simulink model "ctrl_student_HIL103007042017"  (R2015a)
settings: Solver=ode3  StartTime=0.0  StopTime=inf  FixedStep=0.01  RelTol=1e-3
values from neighbouring files (symbols this model uses):
  DesiredPath = 0    [Innput.m]    (also in Input_v3.m = 1)
  Elipscenter_radi = [6 5;0 3 ]    [Innput.m]    (also in Input_v3.m = [3 2;0 1 ])
  eta_dot_ini = [7;0;0]    [Innput.m]    (also in Input_v3.m)
  K = [2;10]    [Input_v3.m]
  K1 = diag([1,1,4])    [Input_v3.m]
  K2 = diag([200,50,3])    [Input_v3.m]    (also in inputDPgains.m = [1 0 0; 0 1 0; 0 0 1])
  l1 = [1 0 0;0 1 0;0 0 0.05]    [Input_v3.m]    (also in inputDPgains.m = [1 0 0; 0 1 0; 0 0 1])
  l2 = [1 0 0;0 1 0;0 0 0.05]    [Input_v3.m]    (also in inputDPgains.m = [1 0 0; 0 1 0; 0 0 1])
  l3 = [1 0 0;0 1 0;0 0 0.05]    [Input_v3.m]    (also in inputDPgains.m = [1 0 0; 0 1 0; 0 0 1])
  LAW = 1    [Innput.m]    (also in Input_v3.m = 0)
  lim = [1.00;-20;6.45/2;-6.45/2]    [Innput.m]    (also in Input_v3.m = [20;-20;9;-9])
  lim_2 = [1.5;-22;7;-7]    [Innput.m]    (also in Input_v3.m = [25;-25;10;-10])
  m = 14.79    [Input_v3.m]    (also in ctrl_student_init.m)
  mu = mu(1)    [Innput.m]    (also in Input_v3.m = 0.001)
  pd = [2 10;0 4]    [Input_v3.m]
  T_initialDP = T_initialDP*100    (= 6000)    [Input_v3.m]
  U_ref = 0.1    [Innput.m]    (also in Input_v3.m)
libraries: simulink x2
(part 3 of 5)

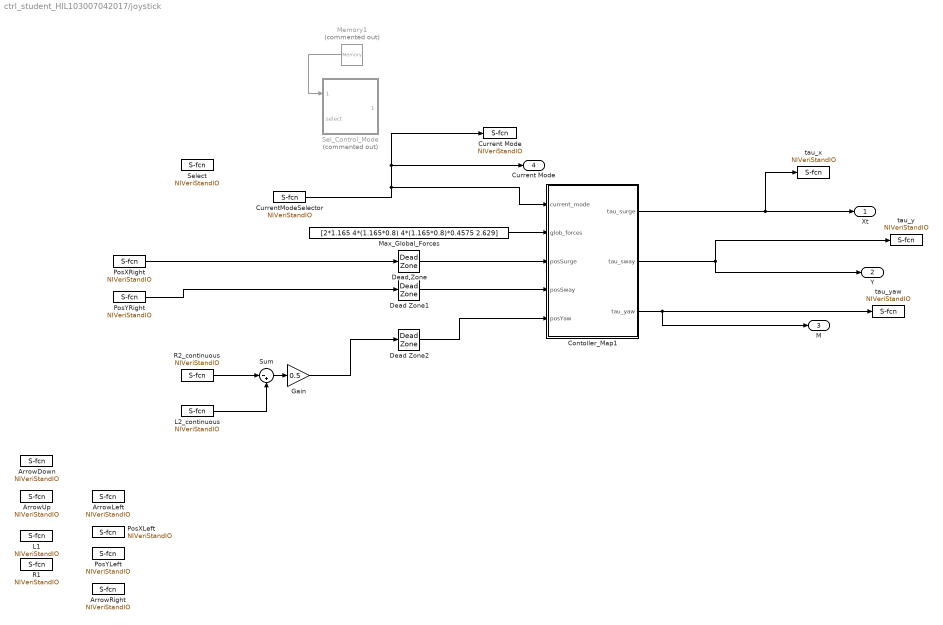
== system ctrl_student_HIL103007042017/joystick ==
  ArrowDown : S-Function  Priority=9  FunctionName=NIVeriStandIO  Parameters=width dtype portnum stime stype btype  mask(NI VeriStand Inport){portnum=9, width=-1, stime=-1, dtype=auto, stype=auto, btype=1}
      mask prompts: portnum "Port number:"; width "Port dimensions (-1 for dynamically sized):"; stime "Sample time (-1 for inherited):"; dtype "Data type:"; stype "Signal type:"; btype "Block type:"
      mask help: Use this inport on any level of nested subsystems to allow NI VeriStand software to map signals to it.
      mask init:
      | NIVeriStandIO_init;
      settings: CopyFcn=NIVeriStand_MDL_functions('', 'IO_copy');  DeleteFcn=NIVeriStand_MDL_functions('', 'IO_delete');  MoveFcn=set_param(gcb, 'Mask', 'on');
      mask Callback portnum: NIVeriStand_MDL_functions('', 'IO_setportnum');
      mask TypeOptions dtype: auto | double | single | int8 | uint8 | int16 | uint16 | int32 | uint32 | boolean
      mask Callback dtype: NIVeriStand_MDL_functions('', 'IO_booleansignal');
      mask TypeOptions stype: auto | real | complex
      mask Display:
      | patch([-x x], [-y y], [.90980 .81960 .32156]);
      | plot([xrad -x x xrad], [yrad -y y yrad]);
      | fprintf('NI In%d', portnum);
  ArrowLeft : S-Function  Priority=11  FunctionName=NIVeriStandIO  Parameters=width dtype portnum stime stype btype  mask(NI VeriStand Inport){portnum=11, width=-1, stime=-1, dtype=auto, stype=auto, btype=1}
      mask prompts: portnum "Port number:"; width "Port dimensions (-1 for dynamically sized):"; stime "Sample time (-1 for inherited):"; dtype "Data type:"; stype "Signal type:"; btype "Block type:"
      mask help: Use this inport on any level of nested subsystems to allow NI VeriStand software to map signals to it.
      mask init:
      | NIVeriStandIO_init;
      settings: CopyFcn=NIVeriStand_MDL_functions('', 'IO_copy');  DeleteFcn=NIVeriStand_MDL_functions('', 'IO_delete');  MoveFcn=set_param(gcb, 'Mask', 'on');
      mask Callback portnum: NIVeriStand_MDL_functions('', 'IO_setportnum');
      mask TypeOptions dtype: auto | double | single | int8 | uint8 | int16 | uint16 | int32 | uint32 | boolean
      mask Callback dtype: NIVeriStand_MDL_functions('', 'IO_booleansignal');
      mask TypeOptions stype: auto | real | complex
      mask Display:
      | patch([-x x], [-y y], [.90980 .81960 .32156]);
      | plot([xrad -x x xrad], [yrad -y y yrad]);
      | fprintf('NI In%d', portnum);
  ArrowRight : S-Function  Priority=12  FunctionName=NIVeriStandIO  Parameters=width dtype portnum stime stype btype  mask(NI VeriStand Inport){portnum=12, width=-1, stime=-1, dtype=auto, stype=auto, btype=1}
      mask prompts: portnum "Port number:"; width "Port dimensions (-1 for dynamically sized):"; stime "Sample time (-1 for inherited):"; dtype "Data type:"; stype "Signal type:"; btype "Block type:"
      mask help: Use this inport on any level of nested subsystems to allow NI VeriStand software to map signals to it.
      mask init:
      | NIVeriStandIO_init;
      settings: CopyFcn=NIVeriStand_MDL_functions('', 'IO_copy');  DeleteFcn=NIVeriStand_MDL_functions('', 'IO_delete');  MoveFcn=set_param(gcb, 'Mask', 'on');
      mask Callback portnum: NIVeriStand_MDL_functions('', 'IO_setportnum');
      mask TypeOptions dtype: auto | double | single | int8 | uint8 | int16 | uint16 | int32 | uint32 | boolean
      mask Callback dtype: NIVeriStand_MDL_functions('', 'IO_booleansignal');
      mask TypeOptions stype: auto | real | complex
      mask Display:
      | patch([-x x], [-y y], [.90980 .81960 .32156]);
      | plot([xrad -x x xrad], [yrad -y y yrad]);
      | fprintf('NI In%d', portnum);
  ArrowUp : S-Function  Priority=10  FunctionName=NIVeriStandIO  Parameters=width dtype portnum stime stype btype  mask(NI VeriStand Inport){portnum=10, width=-1, stime=-1, dtype=auto, stype=auto, btype=1}
      mask prompts: portnum "Port number:"; width "Port dimensions (-1 for dynamically sized):"; stime "Sample time (-1 for inherited):"; dtype "Data type:"; stype "Signal type:"; btype "Block type:"
      mask help: Use this inport on any level of nested subsystems to allow NI VeriStand software to map signals to it.
      mask init:
      | NIVeriStandIO_init;
      settings: CopyFcn=NIVeriStand_MDL_functions('', 'IO_copy');  DeleteFcn=NIVeriStand_MDL_functions('', 'IO_delete');  MoveFcn=set_param(gcb, 'Mask', 'on');
      mask Callback portnum: NIVeriStand_MDL_functions('', 'IO_setportnum');
      mask TypeOptions dtype: auto | double | single | int8 | uint8 | int16 | uint16 | int32 | uint32 | boolean
      mask Callback dtype: NIVeriStand_MDL_functions('', 'IO_booleansignal');
      mask TypeOptions stype: auto | real | complex
      mask Display:
      | patch([-x x], [-y y], [.90980 .81960 .32156]);
      | plot([xrad -x x xrad], [yrad -y y yrad]);
      | fprintf('NI In%d', portnum);
  Contoller_Map1 : MATLAB Function  TreatAsAtomicUnit=on
  "Current Mode " : S-Function  Priority=1  FunctionName=NIVeriStandIO  Parameters=width dtype portnum stime stype btype  mask(NI VeriStand Outport){portnum=1, width=-1, stime=-1, dtype=auto, stype=auto, btype=0}
      mask prompts: portnum "Port number:"; width "Port dimensions (-1 for dynamically sized):"; stime "Sample time (-1 for inherited):"; dtype "Data type:"; stype "Signal type:"; btype "Block type:"
      mask help: Use this outport on any level of nested subsystems to allow NI VeriStand software to map signals to it.
      mask init:
      | NIVeriStandIO_init;
      settings: CopyFcn=NIVeriStand_MDL_functions('', 'IO_copy');  DeleteFcn=NIVeriStand_MDL_functions('', 'IO_delete');  MoveFcn=set_param(gcb, 'Mask', 'on');
      mask Callback portnum: NIVeriStand_MDL_functions('', 'IO_setportnum');
      mask TypeOptions dtype: auto | double | single | int8 | uint8 | int16 | uint16 | int32 | uint32 | boolean
      mask Callback dtype: NIVeriStand_MDL_functions('', 'IO_booleansignal');
      mask TypeOptions stype: auto | real | complex
      mask Display:
      | patch([-x x], [-y y], [.90980 .81960 .32156]);
      | plot([xrad -x x xrad], [yrad -y y yrad]);
      | fprintf('NI Out%d', portnum);
  CurrentModeSelector : S-Function  Priority=14  FunctionName=NIVeriStandIO  Parameters=width dtype portnum stime stype btype  mask(NI VeriStand Inport){portnum=14, width=-1, stime=-1, dtype=auto, stype=auto, btype=1}
      mask prompts: portnum "Port number:"; width "Port dimensions (-1 for dynamically sized):"; stime "Sample time (-1 for inherited):"; dtype "Data type:"; stype "Signal type:"; btype "Block type:"
      mask help: Use this inport on any level of nested subsystems to allow NI VeriStand software to map signals to it.
      mask init:
      | NIVeriStandIO_init;
      settings: CopyFcn=NIVeriStand_MDL_functions('', 'IO_copy');  DeleteFcn=NIVeriStand_MDL_functions('', 'IO_delete');  MoveFcn=set_param(gcb, 'Mask', 'on');
      mask Callback portnum: NIVeriStand_MDL_functions('', 'IO_setportnum');
      mask TypeOptions dtype: auto | double | single | int8 | uint8 | int16 | uint16 | int32 | uint32 | boolean
      mask Callback dtype: NIVeriStand_MDL_functions('', 'IO_booleansignal');
      mask TypeOptions stype: auto | real | complex
      mask Display:
      | patch([-x x], [-y y], [.90980 .81960 .32156]);
      | plot([xrad -x x xrad], [yrad -y y yrad]);
      | fprintf('NI In%d', portnum);
  Dead Zone : DeadZone  LowerValue=-0.05  UpperValue=0.05  SaturateOnIntegerOverflow=on
  Dead Zone1 : DeadZone  LowerValue=-0.05  UpperValue=0.05  SaturateOnIntegerOverflow=on
  Dead Zone2 : DeadZone  LowerValue=-0.05  UpperValue=0.05  SaturateOnIntegerOverflow=on
  Gain : Gain  Gain=0.5
  L1 : S-Function  Priority=7  FunctionName=NIVeriStandIO  Parameters=width dtype portnum stime stype btype  mask(NI VeriStand Inport){portnum=7, width=-1, stime=-1, dtype=auto, stype=auto, btype=1}
      mask prompts: portnum "Port number:"; width "Port dimensions (-1 for dynamically sized):"; stime "Sample time (-1 for inherited):"; dtype "Data type:"; stype "Signal type:"; btype "Block type:"
      mask help: Use this inport on any level of nested subsystems to allow NI VeriStand software to map signals to it.
      mask init:
      | NIVeriStandIO_init;
      settings: CopyFcn=NIVeriStand_MDL_functions('', 'IO_copy');  DeleteFcn=NIVeriStand_MDL_functions('', 'IO_delete');  MoveFcn=set_param(gcb, 'Mask', 'on');
      mask Callback portnum: NIVeriStand_MDL_functions('', 'IO_setportnum');
      mask TypeOptions dtype: auto | double | single | int8 | uint8 | int16 | uint16 | int32 | uint32 | boolean
      mask Callback dtype: NIVeriStand_MDL_functions('', 'IO_booleansignal');
      mask TypeOptions stype: auto | real | complex
      mask Display:
      | patch([-x x], [-y y], [.90980 .81960 .32156]);
      | plot([xrad -x x xrad], [yrad -y y yrad]);
      | fprintf('NI In%d', portnum);
  L2_continuous : S-Function  Priority=1  FunctionName=NIVeriStandIO  Parameters=width dtype portnum stime stype btype  mask(NI VeriStand Inport){portnum=1, width=-1, stime=-1, dtype=auto, stype=auto, btype=1}
      mask prompts: portnum "Port number:"; width "Port dimensions (-1 for dynamically sized):"; stime "Sample time (-1 for inherited):"; dtype "Data type:"; stype "Signal type:"; btype "Block type:"
      mask help: Use this inport on any level of nested subsystems to allow NI VeriStand software to map signals to it.
      mask init:
      | NIVeriStandIO_init;
      settings: CopyFcn=NIVeriStand_MDL_functions('', 'IO_copy');  DeleteFcn=NIVeriStand_MDL_functions('', 'IO_delete');  MoveFcn=set_param(gcb, 'Mask', 'on');
      mask Callback portnum: NIVeriStand_MDL_functions('', 'IO_setportnum');
      mask TypeOptions dtype: auto | double | single | int8 | uint8 | int16 | uint16 | int32 | uint32 | boolean
      mask Callback dtype: NIVeriStand_MDL_functions('', 'IO_booleansignal');
      mask TypeOptions stype: auto | real | complex
      mask Display:
      | patch([-x x], [-y y], [.90980 .81960 .32156]);
      | plot([xrad -x x xrad], [yrad -y y yrad]);
      | fprintf('NI In%d', portnum);
  Max_Global_Forces : Constant  Value=[2*1.165 4*(1.165*0.8) 4*(1.165*0.8)*0.4575 2.629]
  Memory1 : Memory  Commented=on  X0=2
  PosXLeft : S-Function  Priority=5  FunctionName=NIVeriStandIO  Parameters=width dtype portnum stime stype btype  mask(NI VeriStand Inport){portnum=5, width=-1, stime=-1, dtype=auto, stype=auto, btype=1}
      mask prompts: portnum "Port number:"; width "Port dimensions (-1 for dynamically sized):"; stime "Sample time (-1 for inherited):"; dtype "Data type:"; stype "Signal type:"; btype "Block type:"
      mask help: Use this inport on any level of nested subsystems to allow NI VeriStand software to map signals to it.
      mask init:
      | NIVeriStandIO_init;
      settings: CopyFcn=NIVeriStand_MDL_functions('', 'IO_copy');  DeleteFcn=NIVeriStand_MDL_functions('', 'IO_delete');  MoveFcn=set_param(gcb, 'Mask', 'on');
      mask Callback portnum: NIVeriStand_MDL_functions('', 'IO_setportnum');
      mask TypeOptions dtype: auto | double | single | int8 | uint8 | int16 | uint16 | int32 | uint32 | boolean
      mask Callback dtype: NIVeriStand_MDL_functions('', 'IO_booleansignal');
      mask TypeOptions stype: auto | real | complex
      mask Display:
      | patch([-x x], [-y y], [.90980 .81960 .32156]);
      | plot([xrad -x x xrad], [yrad -y y yrad]);
      | fprintf('NI In%d', portnum);
  PosXRight : S-Function  Priority=2  FunctionName=NIVeriStandIO  Parameters=width dtype portnum stime stype btype  mask(NI VeriStand Inport){portnum=2, width=-1, stime=-1, dtype=auto, stype=auto, btype=1}
      mask prompts: portnum "Port number:"; width "Port dimensions (-1 for dynamically sized):"; stime "Sample time (-1 for inherited):"; dtype "Data type:"; stype "Signal type:"; btype "Block type:"
      mask help: Use this inport on any level of nested subsystems to allow NI VeriStand software to map signals to it.
      mask init:
      | NIVeriStandIO_init;
      settings: CopyFcn=NIVeriStand_MDL_functions('', 'IO_copy');  DeleteFcn=NIVeriStand_MDL_functions('', 'IO_delete');  MoveFcn=set_param(gcb, 'Mask', 'on');
      mask Callback portnum: NIVeriStand_MDL_functions('', 'IO_setportnum');
      mask TypeOptions dtype: auto | double | single | int8 | uint8 | int16 | uint16 | int32 | uint32 | boolean
      mask Callback dtype: NIVeriStand_MDL_functions('', 'IO_booleansignal');
      mask TypeOptions stype: auto | real | complex
      mask Display:
      | patch([-x x], [-y y], [.90980 .81960 .32156]);
      | plot([xrad -x x xrad], [yrad -y y yrad]);
      | fprintf('NI In%d', portnum);
  PosYLeft : S-Function  Priority=6  FunctionName=NIVeriStandIO  Parameters=width dtype portnum stime stype btype  mask(NI VeriStand Inport){portnum=6, width=-1, stime=-1, dtype=auto, stype=auto, btype=1}
      mask prompts: portnum "Port number:"; width "Port dimensions (-1 for dynamically sized):"; stime "Sample time (-1 for inherited):"; dtype "Data type:"; stype "Signal type:"; btype "Block type:"
      mask help: Use this inport on any level of nested subsystems to allow NI VeriStand software to map signals to it.
      mask init:
      | NIVeriStandIO_init;
      settings: CopyFcn=NIVeriStand_MDL_functions('', 'IO_copy');  DeleteFcn=NIVeriStand_MDL_functions('', 'IO_delete');  MoveFcn=set_param(gcb, 'Mask', 'on');
      mask Callback portnum: NIVeriStand_MDL_functions('', 'IO_setportnum');
      mask TypeOptions dtype: auto | double | single | int8 | uint8 | int16 | uint16 | int32 | uint32 | boolean
      mask Callback dtype: NIVeriStand_MDL_functions('', 'IO_booleansignal');
      mask TypeOptions stype: auto | real | complex
      mask Display:
      | patch([-x x], [-y y], [.90980 .81960 .32156]);
      | plot([xrad -x x xrad], [yrad -y y yrad]);
      | fprintf('NI In%d', portnum);
  PosYRight : S-Function  Priority=3  FunctionName=NIVeriStandIO  Parameters=width dtype portnum stime stype btype  mask(NI VeriStand Inport){portnum=3, width=-1, stime=-1, dtype=auto, stype=auto, btype=1}
      mask prompts: portnum "Port number:"; width "Port dimensions (-1 for dynamically sized):"; stime "Sample time (-1 for inherited):"; dtype "Data type:"; stype "Signal type:"; btype "Block type:"
      mask help: Use this inport on any level of nested subsystems to allow NI VeriStand software to map signals to it.
      mask init:
      | NIVeriStandIO_init;
      settings: CopyFcn=NIVeriStand_MDL_functions('', 'IO_copy');  DeleteFcn=NIVeriStand_MDL_functions('', 'IO_delete');  MoveFcn=set_param(gcb, 'Mask', 'on');
      mask Callback portnum: NIVeriStand_MDL_functions('', 'IO_setportnum');
      mask TypeOptions dtype: auto | double | single | int8 | uint8 | int16 | uint16 | int32 | uint32 | boolean
      mask Callback dtype: NIVeriStand_MDL_functions('', 'IO_booleansignal');
      mask TypeOptions stype: auto | real | complex
      mask Display:
      | patch([-x x], [-y y], [.90980 .81960 .32156]);
      | plot([xrad -x x xrad], [yrad -y y yrad]);
      | fprintf('NI In%d', portnum);
  R1 : S-Function  Priority=8  FunctionName=NIVeriStandIO  Parameters=width dtype portnum stime stype btype  mask(NI VeriStand Inport){portnum=8, width=-1, stime=-1, dtype=auto, stype=auto, btype=1}
      mask prompts: portnum "Port number:"; width "Port dimensions (-1 for dynamically sized):"; stime "Sample time (-1 for inherited):"; dtype "Data type:"; stype "Signal type:"; btype "Block type:"
      mask help: Use this inport on any level of nested subsystems to allow NI VeriStand software to map signals to it.
      mask init:
      | NIVeriStandIO_init;
      settings: CopyFcn=NIVeriStand_MDL_functions('', 'IO_copy');  DeleteFcn=NIVeriStand_MDL_functions('', 'IO_delete');  MoveFcn=set_param(gcb, 'Mask', 'on');
      mask Callback portnum: NIVeriStand_MDL_functions('', 'IO_setportnum');
      mask TypeOptions dtype: auto | double | single | int8 | uint8 | int16 | uint16 | int32 | uint32 | boolean
      mask Callback dtype: NIVeriStand_MDL_functions('', 'IO_booleansignal');
      mask TypeOptions stype: auto | real | complex
      mask Display:
      | patch([-x x], [-y y], [.90980 .81960 .32156]);
      | plot([xrad -x x xrad], [yrad -y y yrad]);
      | fprintf('NI In%d', portnum);
  R2_continuous : S-Function  Priority=4  FunctionName=NIVeriStandIO  Parameters=width dtype portnum stime stype btype  mask(NI VeriStand Inport){portnum=4, width=-1, stime=-1, dtype=auto, stype=auto, btype=1}
      mask prompts: portnum "Port number:"; width "Port dimensions (-1 for dynamically sized):"; stime "Sample time (-1 for inherited):"; dtype "Data type:"; stype "Signal type:"; btype "Block type:"
      mask help: Use this inport on any level of nested subsystems to allow NI VeriStand software to map signals to it.
      mask init:
      | NIVeriStandIO_init;
      settings: CopyFcn=NIVeriStand_MDL_functions('', 'IO_copy');  DeleteFcn=NIVeriStand_MDL_functions('', 'IO_delete');  MoveFcn=set_param(gcb, 'Mask', 'on');
      mask Callback portnum: NIVeriStand_MDL_functions('', 'IO_setportnum');
      mask TypeOptions dtype: auto | double | single | int8 | uint8 | int16 | uint16 | int32 | uint32 | boolean
      mask Callback dtype: NIVeriStand_MDL_functions('', 'IO_booleansignal');
      mask TypeOptions stype: auto | real | complex
      mask Display:
      | patch([-x x], [-y y], [.90980 .81960 .32156]);
      | plot([xrad -x x xrad], [yrad -y y yrad]);
      | fprintf('NI In%d', portnum);
  Sel_Control_Mode : MATLAB Function  Commented=on  TreatAsAtomicUnit=on
  Select : S-Function  Priority=13  FunctionName=NIVeriStandIO  Parameters=width dtype portnum stime stype btype  mask(NI VeriStand Inport){portnum=13, width=-1, stime=-1, dtype=auto, stype=auto, btype=1}
      mask prompts: portnum "Port number:"; width "Port dimensions (-1 for dynamically sized):"; stime "Sample time (-1 for inherited):"; dtype "Data type:"; stype "Signal type:"; btype "Block type:"
      mask help: Use this inport on any level of nested subsystems to allow NI VeriStand software to map signals to it.
      mask init:
      | NIVeriStandIO_init;
      settings: CopyFcn=NIVeriStand_MDL_functions('', 'IO_copy');  DeleteFcn=NIVeriStand_MDL_functions('', 'IO_delete');  MoveFcn=set_param(gcb, 'Mask', 'on');
      mask Callback portnum: NIVeriStand_MDL_functions('', 'IO_setportnum');
      mask TypeOptions dtype: auto | double | single | int8 | uint8 | int16 | uint16 | int32 | uint32 | boolean
      mask Callback dtype: NIVeriStand_MDL_functions('', 'IO_booleansignal');
      mask TypeOptions stype: auto | real | complex
      mask Display:
      | patch([-x x], [-y y], [.90980 .81960 .32156]);
      | plot([xrad -x x xrad], [yrad -y y yrad]);
      | fprintf('NI In%d', portnum);
  Sum : Sum  Inputs=|-+
  tau_x : S-Function  Priority=3  FunctionName=NIVeriStandIO  Parameters=width dtype portnum stime stype btype  mask(NI VeriStand Outport){portnum=3, width=-1, stime=-1, dtype=auto, stype=auto, btype=0}
      mask prompts: portnum "Port number:"; width "Port dimensions (-1 for dynamically sized):"; stime "Sample time (-1 for inherited):"; dtype "Data type:"; stype "Signal type:"; btype "Block type:"
      mask help: Use this outport on any level of nested subsystems to allow NI VeriStand software to map signals to it.
      mask init:
      | NIVeriStandIO_init;
      settings: CopyFcn=NIVeriStand_MDL_functions('', 'IO_copy');  DeleteFcn=NIVeriStand_MDL_functions('', 'IO_delete');  MoveFcn=set_param(gcb, 'Mask', 'on');
      mask Callback portnum: NIVeriStand_MDL_functions('', 'IO_setportnum');
      mask TypeOptions dtype: auto | double | single | int8 | uint8 | int16 | uint16 | int32 | uint32 | boolean
      mask Callback dtype: NIVeriStand_MDL_functions('', 'IO_booleansignal');
      mask TypeOptions stype: auto | real | complex
      mask Display:
      | patch([-x x], [-y y], [.90980 .81960 .32156]);
      | plot([xrad -x x xrad], [yrad -y y yrad]);
      | fprintf('NI Out%d', portnum);
  tau_y : S-Function  Priority=4  FunctionName=NIVeriStandIO  Parameters=width dtype portnum stime stype btype  mask(NI VeriStand Outport){portnum=4, width=-1, stime=-1, dtype=auto, stype=auto, btype=0}
      mask prompts: portnum "Port number:"; width "Port dimensions (-1 for dynamically sized):"; stime "Sample time (-1 for inherited):"; dtype "Data type:"; stype "Signal type:"; btype "Block type:"
      mask help: Use this outport on any level of nested subsystems to allow NI VeriStand software to map signals to it.
      mask init:
      | NIVeriStandIO_init;
      settings: CopyFcn=NIVeriStand_MDL_functions('', 'IO_copy');  DeleteFcn=NIVeriStand_MDL_functions('', 'IO_delete');  MoveFcn=set_param(gcb, 'Mask', 'on');
      mask Callback portnum: NIVeriStand_MDL_functions('', 'IO_setportnum');
      mask TypeOptions dtype: auto | double | single | int8 | uint8 | int16 | uint16 | int32 | uint32 | boolean
      mask Callback dtype: NIVeriStand_MDL_functions('', 'IO_booleansignal');
      mask TypeOptions stype: auto | real | complex
      mask Display:
      | patch([-x x], [-y y], [.90980 .81960 .32156]);
      | plot([xrad -x x xrad], [yrad -y y yrad]);
      | fprintf('NI Out%d', portnum);
  tau_yaw : S-Function  Priority=2  FunctionName=NIVeriStandIO  Parameters=width dtype portnum stime stype btype  mask(NI VeriStand Outport){portnum=2, width=-1, stime=-1, dtype=auto, stype=auto, btype=0}
      mask prompts: portnum "Port number:"; width "Port dimensions (-1 for dynamically sized):"; stime "Sample time (-1 for inherited):"; dtype "Data type:"; stype "Signal type:"; btype "Block type:"
      mask help: Use this outport on any level of nested subsystems to allow NI VeriStand software to map signals to it.
      mask init:
      | NIVeriStandIO_init;
      settings: CopyFcn=NIVeriStand_MDL_functions('', 'IO_copy');  DeleteFcn=NIVeriStand_MDL_functions('', 'IO_delete');  MoveFcn=set_param(gcb, 'Mask', 'on');
      mask Callback portnum: NIVeriStand_MDL_functions('', 'IO_setportnum');
      mask TypeOptions dtype: auto | double | single | int8 | uint8 | int16 | uint16 | int32 | uint32 | boolean
      mask Callback dtype: NIVeriStand_MDL_functions('', 'IO_booleansignal');
      mask TypeOptions stype: auto | real | complex
      mask Display:
      | patch([-x x], [-y y], [.90980 .81960 .32156]);
      | plot([xrad -x x xrad], [yrad -y y yrad]);
      | fprintf('NI Out%d', portnum);
  Xt : Outport
  Y : Outport  Port=2
  M : Outport  Port=3
  Current Mode : Outport  Port=4
  wires:
  PosXRight/1 -> Dead Zone/1
  PosYRight/1 -> Dead Zone1/1
  Dead Zone/1 -> Contoller_Map1/3(posSurge)
  Dead Zone1/1 -> Contoller_Map1/4(posSway)
  Memory1/1 -> Sel_Control_Mode/1(previous_condition)
  CurrentModeSelector/1 -> "Current Mode "/1, Current Mode/1, Contoller_Map1/1(current_mode)
  Dead Zone2/1 -> Contoller_Map1/5(posYaw)
  Max_Global_Forces/1 -> Contoller_Map1/2(glob_forces)
  Contoller_Map1/1(tau_surge) -> Xt/1, tau_x/1
  Contoller_Map1/2(tau_sway) -> Y/1, tau_y/1
  Contoller_Map1/3(tau_yaw) -> tau_yaw/1, M/1
  L2_continuous/1 -> Sum/2
  Sum/1 -> Gain/1
  R2_continuous/1 -> Sum/1
  Gain/1 -> Dead Zone2/1

== system ctrl_student_HIL103007042017/physics_model ==
  "eta_measure " : Inport
  reset : Inport  Port=2
  tau : Inport  Port=3
  nu : Inport  Port=4
  Integrator : Integrator  ExternalReset=rising  InitialConditionSource=external  InitialCondition=[0 0 0]'
  Integrator1 : Integrator  ExternalReset=rising  InitialConditionSource=external  InitialCondition=[0 0 0]'
  Reshape1 : Reshape  OutputDimensionality=Customize  OutputDimensions=[3,1]
  Reshape3 : Reshape  OutputDimensionality=Customize  OutputDimensions=[3,1]
  kinematics : MATLAB Function  TreatAsAtomicUnit=on
  kinetics : MATLAB Function  TreatAsAtomicUnit=on
  eta : Outport
  wires:
  kinetics/1(nu_dot) -> Integrator/1
  Integrator/1 -> Reshape3/1, kinetics/2(nu)
  kinematics/1(eta_dot) -> Integrator1/1
  reset/1 -> Integrator1/2, Integrator/2
  "eta_measure "/1 -> Integrator1/3
  tau/1 -> kinetics/1(tau)
  Reshape3/1 -> kinematics/1(nu)
  Reshape1/1 -> kinematics/2(eta)
  Integrator1/1 -> eta/1, Reshape1/1
  nu/1 -> Integrator/3

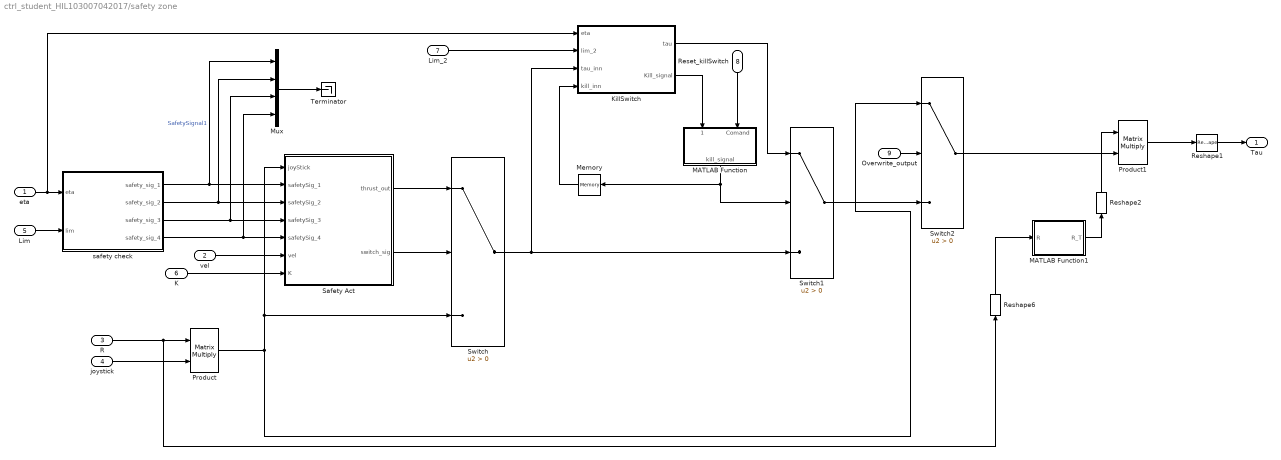
== system ctrl_student_HIL103007042017/safety zone  ==
  eta : Inport
  "vel " : Inport  Port=2
  R : Inport  Port=3
  joystick : Inport  Port=4
  Lim : Inport  Port=5
  K : Inport  Port=6
  Lim_2 : Inport  Port=7
  Reset_killSwitch : Inport  Port=8
  Overwrite_output : Inport  Port=9
  KillSwitch : MATLAB Function  TreatAsAtomicUnit=on
  MATLAB Function : MATLAB Function  TreatAsAtomicUnit=on
  MATLAB Function1 : MATLAB Function  TreatAsAtomicUnit=on
  Memory : Memory
  Mux : Mux
  Product : Product  Multiplication=Matrix(*)
  Product1 : Product  Multiplication=Matrix(*)
  Reshape1 : Reshape  OutputDimensionality=Customize  OutputDimensions=[3,1]
  Reshape2 : Reshape  OutputDimensionality=Customize  OutputDimensions=[3,3]
  Reshape6 : Reshape  OutputDimensionality=Customize  OutputDimensions=[3,3]
  Safety Act : MATLAB Function  TreatAsAtomicUnit=on
  Switch : Switch  Criteria=u2 > Threshold
  Switch1 : Switch  Criteria=u2 > Threshold
  Switch2 : Switch  Criteria=u2 > Threshold
  Terminator : Terminator
  safety check : MATLAB Function  TreatAsAtomicUnit=on
  Tau : Outport
  wires:
  safety check/1(safety_sig_1) -> Mux/1, Safety Act/2(safetySig_1)  "SafetySignal1"
  Safety Act/1(thrust_out) -> Switch/1
  safety check/2(safety_sig_2) -> Mux/2, Safety Act/3(safetySig_2)
  safety check/3(safety_sig_3) -> Safety Act/4(safetySig_3), Mux/3
  safety check/4(safety_sig_4) -> Safety Act/5(safetySig_4), Mux/4
  "vel "/1 -> Safety Act/6(vel)
  Mux/1 -> Terminator/1
  Lim/1 -> safety check/2(lim)
  Safety Act/2(switch_sig) -> Switch/2
  K/1 -> Safety Act/7(K)
  eta/1 -> KillSwitch/1(eta), safety check/1(eta)
  Lim_2/1 -> KillSwitch/2(lim_2)
  Memory/1 -> KillSwitch/4(kill_inn)
  Switch/1 -> KillSwitch/3(tau_inn), Switch1/3
  KillSwitch/1(tau) -> Switch1/1
  MATLAB Function/1(kill_signal) -> Memory/1, Switch1/2
  Reset_killSwitch/1 -> MATLAB Function/2(Comand)
  Overwrite_output/1 -> Switch2/2
  Switch1/1 -> Switch2/3
  KillSwitch/2(Kill_signal) -> MATLAB Function/1(kill_signalInn)
  R/1 -> Reshape6/1, Product/1
  joystick/1 -> Product/2
  Product/1 -> Safety Act/1(joyStick), Switch/3, Switch2/1
  MATLAB Function1/1(R_T) -> Reshape2/1
  Product1/1 -> Reshape1/1
  Reshape1/1 -> Tau/1
  Switch2/1 -> Product1/2
  Reshape6/1 -> MATLAB Function1/1(R)
  Reshape2/1 -> Product1/1

== system ctrl_student_HIL103007042017/tau to CSE mocell (only use for HIL testing) ==
  tau_d to model : Inport
  integrator reset : Inport  Port=2
  Constant1 : Constant  Value=eta_dot_ini
  Demux : Demux  Outputs=3
  Demux1 : Demux  Outputs=3
  N_d : S-Function  Priority=2  FunctionName=NIVeriStandIO  Parameters=width dtype portnum stime stype btype  mask(NI VeriStand Outport){portnum=2, width=-1, stime=-1, dtype=auto, stype=auto, btype=0}
      mask prompts: portnum "Port number:"; width "Port dimensions (-1 for dynamically sized):"; stime "Sample time (-1 for inherited):"; dtype "Data type:"; stype "Signal type:"; btype "Block type:"
      mask help: Use this outport on any level of nested subsystems to allow NI VeriStand software to map signals to it.
      mask init:
      | NIVeriStandIO_init;
      settings: CopyFcn=NIVeriStand_MDL_functions('', 'IO_copy');  DeleteFcn=NIVeriStand_MDL_functions('', 'IO_delete');  MoveFcn=set_param(gcb, 'Mask', 'on');
      mask Callback portnum: NIVeriStand_MDL_functions('', 'IO_setportnum');
      mask TypeOptions dtype: auto | double | single | int8 | uint8 | int16 | uint16 | int32 | uint32 | boolean
      mask Callback dtype: NIVeriStand_MDL_functions('', 'IO_booleansignal');
      mask TypeOptions stype: auto | real | complex
      mask Display:
      | patch([-x x], [-y y], [.90980 .81960 .32156]);
      | plot([xrad -x x xrad], [yrad -y y yrad]);
      | fprintf('NI Out%d', portnum);
  X_d : S-Function  Priority=1  FunctionName=NIVeriStandIO  Parameters=width dtype portnum stime stype btype  mask(NI VeriStand Outport){portnum=1, width=-1, stime=-1, dtype=auto, stype=auto, btype=0}
      mask prompts: portnum "Port number:"; width "Port dimensions (-1 for dynamically sized):"; stime "Sample time (-1 for inherited):"; dtype "Data type:"; stype "Signal type:"; btype "Block type:"
      mask help: Use this outport on any level of nested subsystems to allow NI VeriStand software to map signals to it.
      mask init:
      | NIVeriStandIO_init;
      settings: CopyFcn=NIVeriStand_MDL_functions('', 'IO_copy');  DeleteFcn=NIVeriStand_MDL_functions('', 'IO_delete');  MoveFcn=set_param(gcb, 'Mask', 'on');
      mask Callback portnum: NIVeriStand_MDL_functions('', 'IO_setportnum');
      mask TypeOptions dtype: auto | double | single | int8 | uint8 | int16 | uint16 | int32 | uint32 | boolean
      mask Callback dtype: NIVeriStand_MDL_functions('', 'IO_booleansignal');
      mask TypeOptions stype: auto | real | complex
      mask Display:
      | patch([-x x], [-y y], [.90980 .81960 .32156]);
      | plot([xrad -x x xrad], [yrad -y y yrad]);
      | fprintf('NI Out%d', portnum);
  Y_d : S-Function  Priority=3  FunctionName=NIVeriStandIO  Parameters=width dtype portnum stime stype btype  mask(NI VeriStand Outport){portnum=3, width=-1, stime=-1, dtype=auto, stype=auto, btype=0}
      mask prompts: portnum "Port number:"; width "Port dimensions (-1 for dynamically sized):"; stime "Sample time (-1 for inherited):"; dtype "Data type:"; stype "Signal type:"; btype "Block type:"
      mask help: Use this outport on any level of nested subsystems to allow NI VeriStand software to map signals to it.
      mask init:
      | NIVeriStandIO_init;
      settings: CopyFcn=NIVeriStand_MDL_functions('', 'IO_copy');  DeleteFcn=NIVeriStand_MDL_functions('', 'IO_delete');  MoveFcn=set_param(gcb, 'Mask', 'on');
      mask Callback portnum: NIVeriStand_MDL_functions('', 'IO_setportnum');
      mask TypeOptions dtype: auto | double | single | int8 | uint8 | int16 | uint16 | int32 | uint32 | boolean
      mask Callback dtype: NIVeriStand_MDL_functions('', 'IO_booleansignal');
      mask TypeOptions stype: auto | real | complex
      mask Display:
      | patch([-x x], [-y y], [.90980 .81960 .32156]);
      | plot([xrad -x x xrad], [yrad -y y yrad]);
      | fprintf('NI Out%d', portnum);
  integrator reset model : S-Function  Priority=7  FunctionName=NIVeriStandIO  Parameters=width dtype portnum stime stype btype  mask(NI VeriStand Outport){portnum=7, width=-1, stime=-1, dtype=auto, stype=auto, btype=0}
      mask prompts: portnum "Port number:"; width "Port dimensions (-1 for dynamically sized):"; stime "Sample time (-1 for inherited):"; dtype "Data type:"; stype "Signal type:"; btype "Block type:"
      mask help: Use this outport on any level of nested subsystems to allow NI VeriStand software to map signals to it.
      mask init:
      | NIVeriStandIO_init;
      settings: CopyFcn=NIVeriStand_MDL_functions('', 'IO_copy');  DeleteFcn=NIVeriStand_MDL_functions('', 'IO_delete');  MoveFcn=set_param(gcb, 'Mask', 'on');
      mask Callback portnum: NIVeriStand_MDL_functions('', 'IO_setportnum');
      mask TypeOptions dtype: auto | double | single | int8 | uint8 | int16 | uint16 | int32 | uint32 | boolean
      mask Callback dtype: NIVeriStand_MDL_functions('', 'IO_booleansignal');
      mask TypeOptions stype: auto | real | complex
      mask Display:
      | patch([-x x], [-y y], [.90980 .81960 .32156]);
      | plot([xrad -x x xrad], [yrad -y y yrad]);
      | fprintf('NI Out%d', portnum);
  "psi_0 " : S-Function  Priority=4  FunctionName=NIVeriStandIO  Parameters=width dtype portnum stime stype btype  mask(NI VeriStand Outport){portnum=4, width=-1, stime=-1, dtype=auto, stype=auto, btype=0}
      mask prompts: portnum "Port number:"; width "Port dimensions (-1 for dynamically sized):"; stime "Sample time (-1 for inherited):"; dtype "Data type:"; stype "Signal type:"; btype "Block type:"
      mask help: Use this outport on any level of nested subsystems to allow NI VeriStand software to map signals to it.
      mask init:
      | NIVeriStandIO_init;
      settings: CopyFcn=NIVeriStand_MDL_functions('', 'IO_copy');  DeleteFcn=NIVeriStand_MDL_functions('', 'IO_delete');  MoveFcn=set_param(gcb, 'Mask', 'on');
      mask Callback portnum: NIVeriStand_MDL_functions('', 'IO_setportnum');
      mask TypeOptions dtype: auto | double | single | int8 | uint8 | int16 | uint16 | int32 | uint32 | boolean
      mask Callback dtype: NIVeriStand_MDL_functions('', 'IO_booleansignal');
      mask TypeOptions stype: auto | real | complex
      mask Display:
      | patch([-x x], [-y y], [.90980 .81960 .32156]);
      | plot([xrad -x x xrad], [yrad -y y yrad]);
      | fprintf('NI Out%d', portnum);
  x_0 : S-Function  Priority=5  FunctionName=NIVeriStandIO  Parameters=width dtype portnum stime stype btype  mask(NI VeriStand Outport){portnum=5, width=-1, stime=-1, dtype=auto, stype=auto, btype=0}
      mask prompts: portnum "Port number:"; width "Port dimensions (-1 for dynamically sized):"; stime "Sample time (-1 for inherited):"; dtype "Data type:"; stype "Signal type:"; btype "Block type:"
      mask help: Use this outport on any level of nested subsystems to allow NI VeriStand software to map signals to it.
      mask init:
      | NIVeriStandIO_init;
      settings: CopyFcn=NIVeriStand_MDL_functions('', 'IO_copy');  DeleteFcn=NIVeriStand_MDL_functions('', 'IO_delete');  MoveFcn=set_param(gcb, 'Mask', 'on');
      mask Callback portnum: NIVeriStand_MDL_functions('', 'IO_setportnum');
      mask TypeOptions dtype: auto | double | single | int8 | uint8 | int16 | uint16 | int32 | uint32 | boolean
      mask Callback dtype: NIVeriStand_MDL_functions('', 'IO_booleansignal');
      mask TypeOptions stype: auto | real | complex
      mask Display:
      | patch([-x x], [-y y], [.90980 .81960 .32156]);
      | plot([xrad -x x xrad], [yrad -y y yrad]);
      | fprintf('NI Out%d', portnum);
  y_0 : S-Function  Priority=6  FunctionName=NIVeriStandIO  Parameters=width dtype portnum stime stype btype  mask(NI VeriStand Outport){portnum=6, width=-1, stime=-1, dtype=auto, stype=auto, btype=0}
      mask prompts: portnum "Port number:"; width "Port dimensions (-1 for dynamically sized):"; stime "Sample time (-1 for inherited):"; dtype "Data type:"; stype "Signal type:"; btype "Block type:"
      mask help: Use this outport on any level of nested subsystems to allow NI VeriStand software to map signals to it.
      mask init:
      | NIVeriStandIO_init;
      settings: CopyFcn=NIVeriStand_MDL_functions('', 'IO_copy');  DeleteFcn=NIVeriStand_MDL_functions('', 'IO_delete');  MoveFcn=set_param(gcb, 'Mask', 'on');
      mask Callback portnum: NIVeriStand_MDL_functions('', 'IO_setportnum');
      mask TypeOptions dtype: auto | double | single | int8 | uint8 | int16 | uint16 | int32 | uint32 | boolean
      mask Callback dtype: NIVeriStand_MDL_functions('', 'IO_booleansignal');
      mask TypeOptions stype: auto | real | complex
      mask Display:
      | patch([-x x], [-y y], [.90980 .81960 .32156]);
      | plot([xrad -x x xrad], [yrad -y y yrad]);
      | fprintf('NI Out%d', portnum);
  wires:
  tau_d to model/1 -> Demux/1
  Demux/1 -> X_d/1
  Demux/2 -> Y_d/1
  Demux/3 -> N_d/1
  integrator reset/1 -> integrator reset model/1
  Constant1/1 -> Demux1/1
  Demux1/2 -> y_0/1
  Demux1/3 -> "psi_0 "/1
  Demux1/1 -> x_0/1

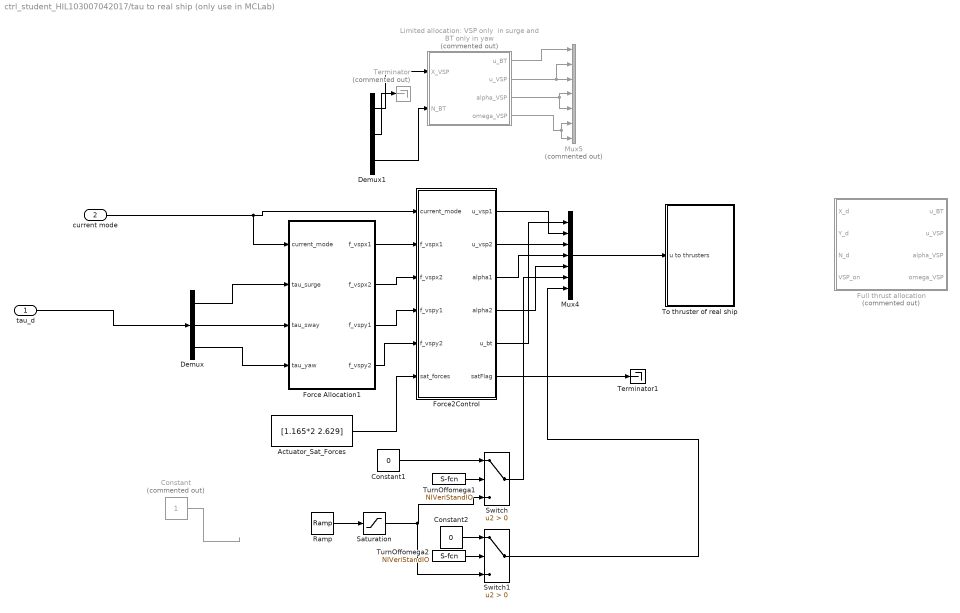
== system ctrl_student_HIL103007042017/tau to real ship (only use in MCLab) ==
  tau_d : Inport
  current mode : Inport  Port=2
  Actuator_Sat_Forces : Constant  Value=[1.165*2 2.629]
  Constant : Constant  Commented=on
  Constant1 : Constant  Value=0
  Constant2 : Constant  Value=0
  Demux : Demux  Outputs=3
  Demux1 : Demux  Outputs=3
  Force Allocation1 : MATLAB Function  TreatAsAtomicUnit=on
  Force2Control : MATLAB Function  TreatAsAtomicUnit=on
  Full thrust allocation : MATLAB Function  Commented=on  TreatAsAtomicUnit=on
  Limited allocation: VSP only  in surge and BT only in yaw : MATLAB Function  Commented=on  TreatAsAtomicUnit=on
  Mux4 : Mux  Inputs=7
  Mux5 : Mux  Commented=on  Inputs=7
  Ramp : simulink/Sources/Ramp  slope=0.1  start=0  X0=0
  Saturation : Saturate  UpperLimit=0.3  LowerLimit=0
  Switch : Switch  Criteria=u2 > Threshold
  Switch1 : Switch  Criteria=u2 > Threshold
  Terminator : Terminator  Commented=on
  Terminator1 : Terminator
  To thruster of real ship : Subsystem
  TurnOffomega1 : S-Function  Priority=1  FunctionName=NIVeriStandIO  Parameters=width dtype portnum stime stype btype  mask(NI VeriStand Inport){portnum=1, width=-1, stime=-1, dtype=auto, stype=auto, btype=1}
      mask prompts: portnum "Port number:"; width "Port dimensions (-1 for dynamically sized):"; stime "Sample time (-1 for inherited):"; dtype "Data type:"; stype "Signal type:"; btype "Block type:"
      mask help: Use this inport on any level of nested subsystems to allow NI VeriStand software to map signals to it.
      mask init:
      | NIVeriStandIO_init;
      settings: CopyFcn=NIVeriStand_MDL_functions('', 'IO_copy');  DeleteFcn=NIVeriStand_MDL_functions('', 'IO_delete');  MoveFcn=set_param(gcb, 'Mask', 'on');
      mask Callback portnum: NIVeriStand_MDL_functions('', 'IO_setportnum');
      mask TypeOptions dtype: auto | double | single | int8 | uint8 | int16 | uint16 | int32 | uint32 | boolean
      mask Callback dtype: NIVeriStand_MDL_functions('', 'IO_booleansignal');
      mask TypeOptions stype: auto | real | complex
      mask Display:
      | patch([-x x], [-y y], [.90980 .81960 .32156]);
      | plot([xrad -x x xrad], [yrad -y y yrad]);
      | fprintf('NI In%d', portnum);
  TurnOffomega2 : S-Function  Priority=2  FunctionName=NIVeriStandIO  Parameters=width dtype portnum stime stype btype  mask(NI VeriStand Inport){portnum=2, width=-1, stime=-1, dtype=auto, stype=auto, btype=1}
      mask prompts: portnum "Port number:"; width "Port dimensions (-1 for dynamically sized):"; stime "Sample time (-1 for inherited):"; dtype "Data type:"; stype "Signal type:"; btype "Block type:"
      mask help: Use this inport on any level of nested subsystems to allow NI VeriStand software to map signals to it.
      mask init:
      | NIVeriStandIO_init;
      settings: CopyFcn=NIVeriStand_MDL_functions('', 'IO_copy');  DeleteFcn=NIVeriStand_MDL_functions('', 'IO_delete');  MoveFcn=set_param(gcb, 'Mask', 'on');
      mask Callback portnum: NIVeriStand_MDL_functions('', 'IO_setportnum');
      mask TypeOptions dtype: auto | double | single | int8 | uint8 | int16 | uint16 | int32 | uint32 | boolean
      mask Callback dtype: NIVeriStand_MDL_functions('', 'IO_booleansignal');
      mask TypeOptions stype: auto | real | complex
      mask Display:
      | patch([-x x], [-y y], [.90980 .81960 .32156]);
      | plot([xrad -x x xrad], [yrad -y y yrad]);
      | fprintf('NI In%d', portnum);
  wires:
  Demux1/1 -> Limited allocation: VSP only  in surge and BT only in yaw/1(X_VSP)
  Demux1/3 -> Limited allocation: VSP only  in surge and BT only in yaw/2(N_BT)
  Demux1/2 -> Terminator/1
  Limited allocation: VSP only  in surge and BT only in yaw/2(u_VSP) -> Mux5/2, Mux5/3
  Constant/1 -> ?
  Limited allocation: VSP only  in surge and BT only in yaw/1(u_BT) -> Mux5/1
  Limited allocation: VSP only  in surge and BT only in yaw/3(alpha_VSP) -> Mux5/4, Mux5/5
  Limited allocation: VSP only  in surge and BT only in yaw/4(omega_VSP) -> Mux5/6, Mux5/7
  Mux4/1 -> To thruster of real ship/1(u to thrusters)
  tau_d/1 -> Demux/1
  Force Allocation1/1(f_vspx1) -> Force2Control/2(f_vspx1)
  Force Allocation1/3(f_vspy1) -> Force2Control/4(f_vspy1)
  Force Allocation1/4(f_vspy2) -> Force2Control/5(f_vspy2)
  Force2Control/1(u_vsp1) -> Mux4/2
  Force2Control/2(u_vsp2) -> Mux4/3
  Force2Control/3(alpha1) -> Mux4/4
  Force2Control/4(alpha2) -> Mux4/5
  Force2Control/5(u_bt) -> Mux4/1
  Force Allocation1/2(f_vspx2) -> Force2Control/3(f_vspx2)
  Ramp/1 -> Saturation/1
  Saturation/1 -> Switch1/3, Switch/3
  TurnOffomega1/1 -> Switch/2
  Switch/1 -> Mux4/6
  TurnOffomega2/1 -> Switch1/2
  Constant2/1 -> Switch1/1
  Switch1/1 -> Mux4/7
  current mode/1 -> Force Allocation1/1(current_mode), Force2Control/1(current_mode)
  Demux/1 -> Force Allocation1/2(tau_surge)
  Demux/2 -> Force Allocation1/3(tau_sway)
  Demux/3 -> Force Allocation1/4(tau_yaw)
  Actuator_Sat_Forces/1 -> Force2Control/6(sat_forces)
  Constant1/1 -> Switch/1
  Force2Control/6(satFlag) -> Terminator1/1

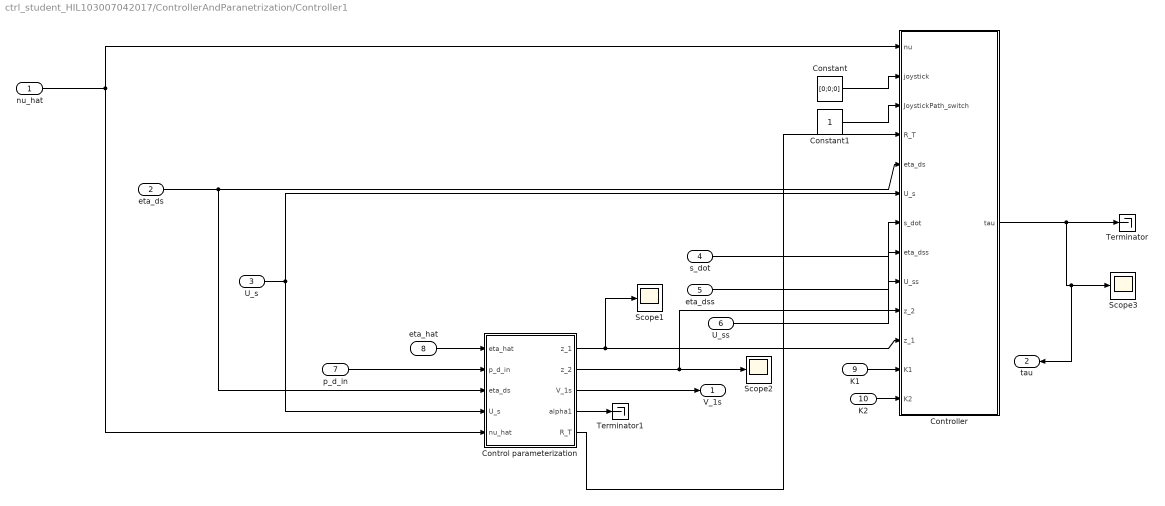
== system ctrl_student_HIL103007042017/ControllerAndParanetrization/Controller1 ==
  nu_hat : Inport
  "eta_ds " : Inport  Port=2
  U_s : Inport  Port=3
  s_dot : Inport  Port=4
  eta_dss : Inport  Port=5
  U_ss : Inport  Port=6
  p_d_in : Inport  Port=7
  eta_hat : Inport  Port=8
  K1 : Inport  Port=9
  K2 : Inport  Port=10
  Constant : Constant  Value=[0;0;0]
  Constant1 : Constant
  Control parameterization : Subsystem
  Controller : Subsystem
  Scope1 : Scope
      settings: YMin=-6.76763  YMax=7.09799  SaveName=ScopeData8
  Scope2 : Scope
  Scope3 : Scope
      settings: YMin=-11.79233  YMax=2.58486  SaveName=ScopeData3
  Terminator : Terminator
  Terminator1 : Terminator
  "V_1s " : Outport
  tau : Outport  Port=2
  wires:
  Control parameterization/1(z_1) -> Scope1/1, Controller/11(z_1)
  Control parameterization/2(z_2) -> Scope2/1, Controller/10(z_2)
  nu_hat/1 -> Controller/1(" nu"), Control parameterization/5(nu_hat)
  Control parameterization/5("R_T ") -> Controller/4(R_T)
  Constant/1 -> Controller/2(joystick)
  Constant1/1 -> Controller/3(JoystickPath_switch)
  Controller/1(tau) -> tau/1, Scope3/1, Terminator/1
  Control parameterization/4(alpha1) -> Terminator1/1
  U_ss/1 -> Controller/9(U_ss)
  s_dot/1 -> Controller/7(s_dot)
  eta_dss/1 -> Controller/8(eta_dss)
  Control parameterization/3("V_1s ") -> "V_1s "/1
  U_s/1 -> Controller/6(U_s), Control parameterization/4(U_s)
  "eta_ds "/1 -> Control parameterization/3("eta_ds "), Controller/5(eta_ds)
  p_d_in/1 -> Control parameterization/2("p_d_in ")
  eta_hat/1 -> Control parameterization/1(eta_hat)
  K1/1 -> Controller/12(K1)
  K2/1 -> Controller/13(K2)

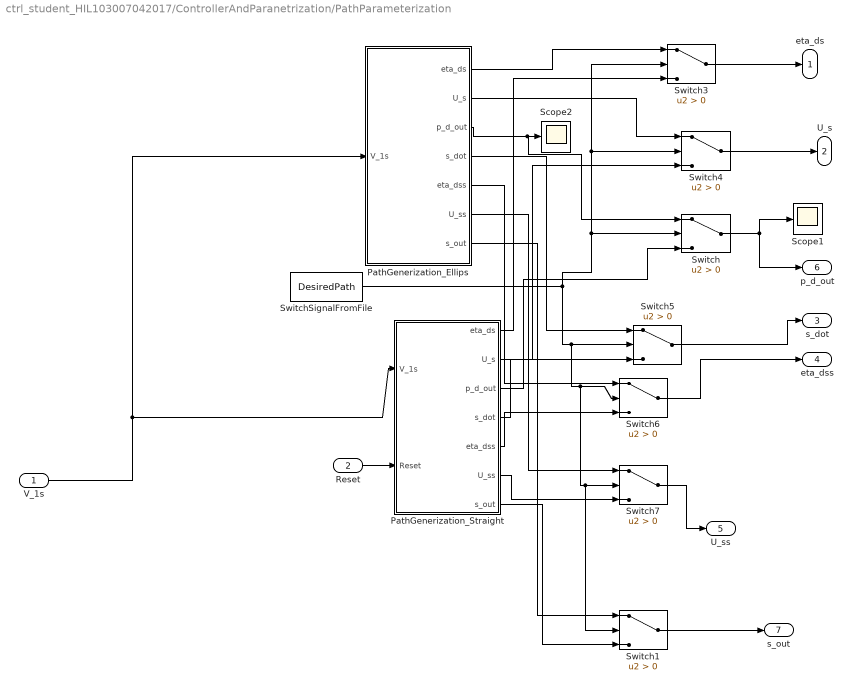
== system ctrl_student_HIL103007042017/ControllerAndParanetrization/PathParameterization ==
  V_1s : Inport
  "Reset " : Inport  Port=2
  PathGenerization_Ellips : Subsystem
  PathGenerization_Straight : Subsystem
  Scope1 : Scope
      settings: YMin=-1.25  YMax=11.25  SaveName=ScopeData2
  Scope2 : Scope
      settings: YMin=-4.75  YMax=12.75  SaveName=ScopeData12
  Switch{,1,3..7} (7 alike) : Switch  Criteria=u2 > Threshold
  SwitchSignalFromFile : Constant  Value=DesiredPath
  eta_ds : Outport
  U_s : Outport  Port=2
  s_dot : Outport  Port=3
  eta_dss : Outport  Port=4
  U_ss : Outport  Port=5
  p_d_out : Outport  Port=6
  s_out : Outport  Port=7
  wires:
  PathGenerization_Ellips/4(s_dot) -> Switch5/1
  PathGenerization_Straight/4(s_dot) -> Switch5/3
  PathGenerization_Ellips/6(U_ss) -> Switch7/1
  PathGenerization_Straight/6(U_ss) -> Switch7/3
  PathGenerization_Straight/5("eta_dss ") -> Switch6/3
  PathGenerization_Straight/1(eta_ds) -> Switch3/3
  PathGenerization_Ellips/1(eta_ds) -> Switch3/1
  PathGenerization_Straight/2(U_s) -> Switch4/3
  PathGenerization_Straight/3(p_d_out) -> Switch/3
  PathGenerization_Ellips/2(U_s) -> Switch4/1
  PathGenerization_Ellips/3(p_d_out) -> Switch/1, Scope2/1
  SwitchSignalFromFile/1 -> Switch4/2, Switch3/2, Switch/2, Switch1/2, Switch7/2, Switch6/2, Switch5/2
  Switch3/1 -> eta_ds/1
  Switch4/1 -> U_s/1
  Switch5/1 -> s_dot/1
  Switch6/1 -> eta_dss/1
  Switch7/1 -> U_ss/1
  V_1s/1 -> PathGenerization_Ellips/1(V_1s), PathGenerization_Straight/1(V_1s)
  Switch/1 -> p_d_out/1, Scope1/1
  PathGenerization_Ellips/5("eta_dss ") -> Switch6/1
  "Reset "/1 -> PathGenerization_Straight/2("Reset ")
  PathGenerization_Straight/7(s_out) -> Switch1/3
  Switch1/1 -> s_out/1
  PathGenerization_Ellips/7(s_out) -> Switch1/1

== system ctrl_student_HIL103007042017/DPObserver1/Bias ==
  eta : Inport
  etaHat : Inport  Port=2
  L3 : Inport  Port=3
  biasOffset : Inport  Port=4  PortDimensions=1
  Constant : Constant  Value=[1;1;1]
  IC1 : InitialCondition  Value=[0;0;0]
  Product : Product
  Reshape1 : Reshape  OutputDimensionality=Customize  OutputDimensions=[3,1]
  Sum : Sum  Inputs=|++
  bHat : Integrator
  bHatDot : MATLAB Function  TreatAsAtomicUnit=on
  bias : Outport
  wires:
  bHatDot/1(bHatDot) -> bHat/1
  eta/1 -> bHatDot/2(eta)
  etaHat/1 -> bHatDot/3(etaHat)
  L3/1 -> bHatDot/1(L3)
  IC1/1 -> bias/1
  Sum/1 -> IC1/1
  biasOffset/1 -> Product/1
  Product/1 -> Reshape1/1
  Constant/1 -> Product/2
  bHat/1 -> Sum/1
  Reshape1/1 -> Sum/2

== system ctrl_student_HIL103007042017/DPObserver1/Subsystem ==
  bHat : Inport
  D : Inport  Port=2
  tau : Inport  Port=3
  eta : Inport  Port=4
  etaHat : Inport  Port=5
  R : Inport  Port=6
  L2 : Inport  Port=7
  IC : InitialCondition  Value=[0;0;0]
  M : MATLAB Function  TreatAsAtomicUnit=on
  nuHat : Integrator  InitialCondition=[0;0;0]
  nuHatDot : MATLAB Function  TreatAsAtomicUnit=on
  nu : Outport
  wires:
  tau/1 -> nuHatDot/6(tau)
  bHat/1 -> nuHatDot/2(bHat)
  M/1(M) -> nuHatDot/4(M)
  nuHat/1 -> nuHatDot/1(nuHat), nu/1
  etaHat/1 -> nuHatDot/9(etaHat)
  R/1 -> nuHatDot/8(R)
  eta/1 -> nuHatDot/7(eta)
  nuHatDot/1(nuHatDot) -> IC/1
  D/1 -> nuHatDot/3(D)
  L2/1 -> nuHatDot/5(L2)
  IC/1 -> nuHat/1

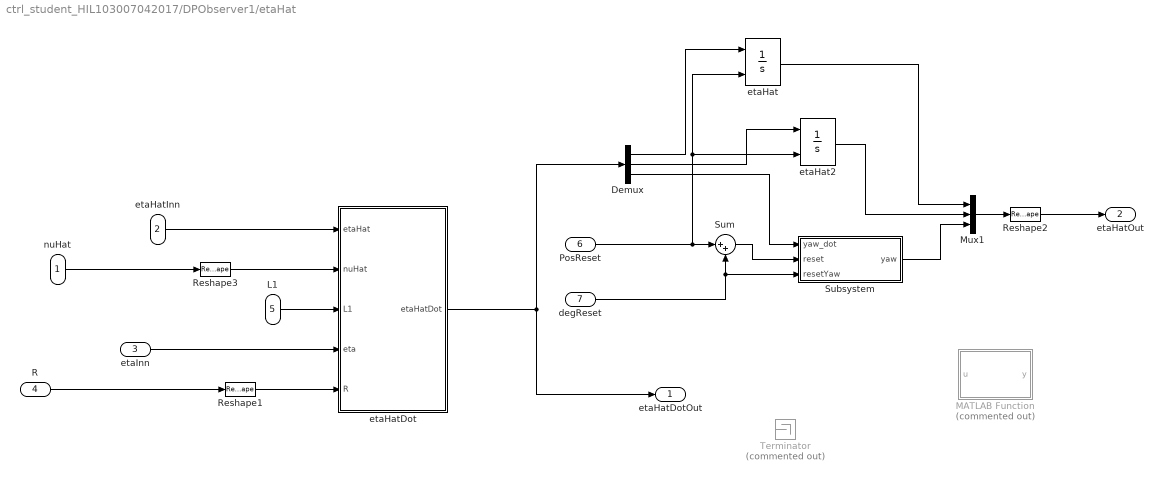
== system ctrl_student_HIL103007042017/DPObserver1/etaHat ==
  nuHat : Inport
  etaHatInn : Inport  Port=2
  etaInn : Inport  Port=3
  R : Inport  Port=4
  L1 : Inport  Port=5
  PosReset : Inport  Port=6
  degReset : Inport  Port=7
  Demux : Demux  Outputs=3
  MATLAB Function : MATLAB Function  Commented=on  TreatAsAtomicUnit=on
  Mux1 : Mux  Inputs=3
  Reshape1 : Reshape  OutputDimensionality=Customize  OutputDimensions=[3,3]
  Reshape2 : Reshape  OutputDimensionality=Customize  OutputDimensions=[3,1]
  Reshape3 : Reshape  OutputDimensionality=Customize  OutputDimensions=[3,1]
  Subsystem : Subsystem
  Sum : Sum  Inputs=|++
  Terminator : Terminator  Commented=on
  etaHat : Integrator  ExternalReset=rising
  etaHat2 : Integrator  ExternalReset=rising
  etaHatDot : MATLAB Function  TreatAsAtomicUnit=on
  etaHatDotOut : Outport
  etaHatOut : Outport  Port=2
  wires:
  etaHatDot/1(etaHatDot) -> Demux/1, etaHatDotOut/1
  L1/1 -> etaHatDot/3(L1)
  R/1 -> Reshape1/1
  nuHat/1 -> Reshape3/1
  etaInn/1 -> etaHatDot/4(eta)
  etaHatInn/1 -> etaHatDot/1(etaHat)
  Reshape3/1 -> etaHatDot/2(nuHat)
  Reshape1/1 -> etaHatDot/5(R)
  Demux/2 -> etaHat2/1
  Demux/1 -> etaHat/1
  Mux1/1 -> Reshape2/1
  Reshape2/1 -> etaHatOut/1
  etaHat/1 -> Mux1/1
  etaHat2/1 -> Mux1/2
  PosReset/1 -> Sum/1, etaHat/2, etaHat2/2
  degReset/1 -> Subsystem/3(resetYaw), Sum/2
  Subsystem/1(yaw) -> Mux1/3
  Demux/3 -> Subsystem/1(yaw_dot)
  Sum/1 -> Subsystem/2(reset)

== system ctrl_student_HIL103007042017/Noise generator/Downsample	signal ==
  sampling frequency : Inport
  step size : Inport  Port=2
  MATLAB Function : MATLAB Function  TreatAsAtomicUnit=on
  counter : Memory
  trigger : Outport
  wires:
  sampling frequency/1 -> MATLAB Function/1(f)
  step size/1 -> MATLAB Function/2(h)
  counter/1 -> MATLAB Function/3(i)
  MATLAB Function/1(count) -> counter/1, trigger/1

== system ctrl_student_HIL103007042017/Noise generator/Sample & hold ==
  trigger : Inport
  input : Inport  Port=2
  Hold : Memory
  MATLAB Function1 : MATLAB Function  TreatAsAtomicUnit=on
  output : Outport
  wires:
  MATLAB Function1/1(output) -> output/1, Hold/1
  trigger/1 -> MATLAB Function1/1(counter)
  input/1 -> MATLAB Function1/2(input)
  Hold/1 -> MATLAB Function1/3(hold)

== system ctrl_student_HIL103007042017/Noise generator/noise generator ==
  step size : Inport
  noise power position : Inport  Port=2
  noise power heading : Inport  Port=3
  Band-limited white noise psi : Subsystem
  Band-limited white noise x : Subsystem
  Band-limited white noise y : Subsystem
  Mux1 : Mux  Inputs=3
  Out1 : Outport
  wires:
  Mux1/1 -> Out1/1
  step size/1 -> Band-limited white noise x/1(step size), Band-limited white noise psi/1(step size), Band-limited white noise y/1(step size)
  noise power position/1 -> Band-limited white noise y/2(power), Band-limited white noise x/2(power)
  Band-limited white noise x/1(noise) -> Mux1/1
  Band-limited white noise y/1(noise) -> Mux1/2
  Band-limited white noise psi/1(noise) -> Mux1/3
  noise power heading/1 -> Band-limited white noise psi/2(power)
